simulink model "model"  (R2021a)
settings: Solver=VariableStepAuto  StartTime=0.0  StopTime=10.0  RelTol=1e-3
values from neighbouring files (symbols this model uses):
  A = [0      1              0           0 ... (first row only)    [modelling.m]
  B = [     0 ... (first row only)    [modelling.m]
  C = [1 0 0 0]    [modelling.m]
  K_lqr = lqr(A,B,qq,R)    [modelling.m]
  X0 = [0; 5*pi/180; 0;0]    [modelling.m]
settings Model: Creator=samlo  LastModifiedBy=samlo

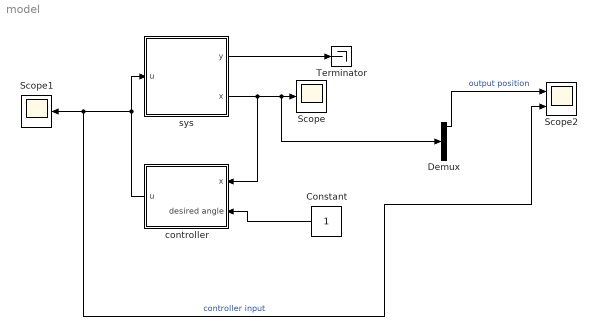
== system model ==
  Constant : Constant
  Demux : Demux
  Scope : Scope
  Scope1 : Scope
  Scope2 : Scope  NumInputPorts=2
  Terminator : Terminator
  controller : Subsystem
  sys : Subsystem
  wires:
  sys/2(x) -> controller/1(x), Demux/1, Scope/1
  sys/1(y) -> Terminator/1
  controller/1(u) -> Scope2/2, Scope1/1, sys/1(u)  "controller input"
  Constant/1 -> controller/2(desired angle)
  Demux/1 -> Scope2/1  "output position"

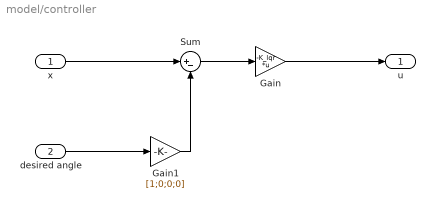
== system model/controller ==
  x : Inport
  desired angle : Inport  Port=2
  Gain : Gain  Gain=-K_lqr  Multiplication=Matrix(K*u)
  Gain1 : Gain  Gain=[1;0;0;0]
  Sum : Sum  Inputs=|+-
  u : Outport
  wires:
  Gain/1 -> u/1
  Gain1/1 -> Sum/2
  x/1 -> Sum/1
  Sum/1 -> Gain/1
  desired angle/1 -> Gain1/1

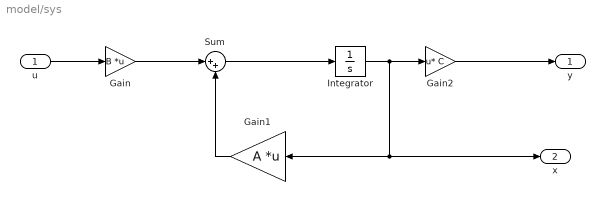
== system model/sys ==
  u : Inport
  Gain : Gain  Gain=B  Multiplication=Matrix(K*u)
  Gain1 : Gain  Gain=A  Multiplication=Matrix(K*u) (u vector)
  Gain2 : Gain  Gain=C  Multiplication=Matrix(u*K)
  Integrator : Integrator  InitialCondition=X0
  Sum : Sum  Inputs=|++
  y : Outport
  x : Outport  Port=2
  wires:
  Sum/1 -> Integrator/1
  Gain/1 -> Sum/1
  Integrator/1 -> Gain2/1, x/1, Gain1/1
  Gain2/1 -> y/1
  Gain1/1 -> Sum/2
  u/1 -> Gain/1
